simulink model "Power_Control"  (R2023b)
settings: Solver=FixedStepAuto  StartTime=0.0  StopTime=0.225  RelTol=1e-3
libraries: simulink x1
settings Model: Creator=no  LastModifiedBy=joser
settings OptimizationCC: DefaultParameterBehavior=Inlined
settings RTWCC: Description=INTECRIO Real-Time Target  SystemTargetFile=irt.tlc  TemplateMakefile=irt_default_tmf
settings STFCustomTargetCC: UtilityFuncGeneration=Shared location  MatFileLogging=on  GRTInterface=on  SystemTargetFile=irt.tlc
settings GRTTargetCC: UtilityFuncGeneration=Shared location  ParMdlRefBuildCompliant=off  CompOptLevelCompliant=off  ConcurrentExecutionCompliant=off  CombineOutputUpdateFcns=off  CPPClassGenCompliant=off  GRTInterface=on  UseToolchainInfoCompliant=off  GenerateASAP2=on

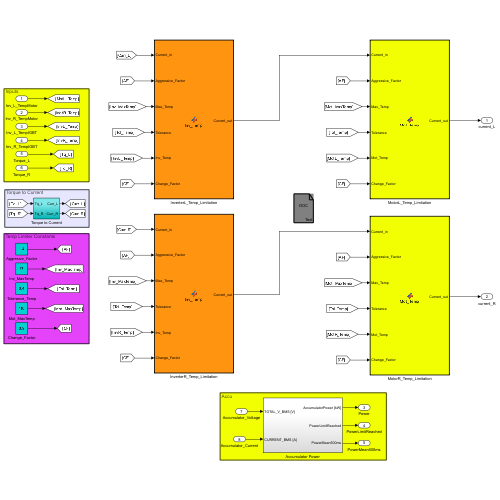
[thumbnail: Simulink's stored preview of the top-level diagram]
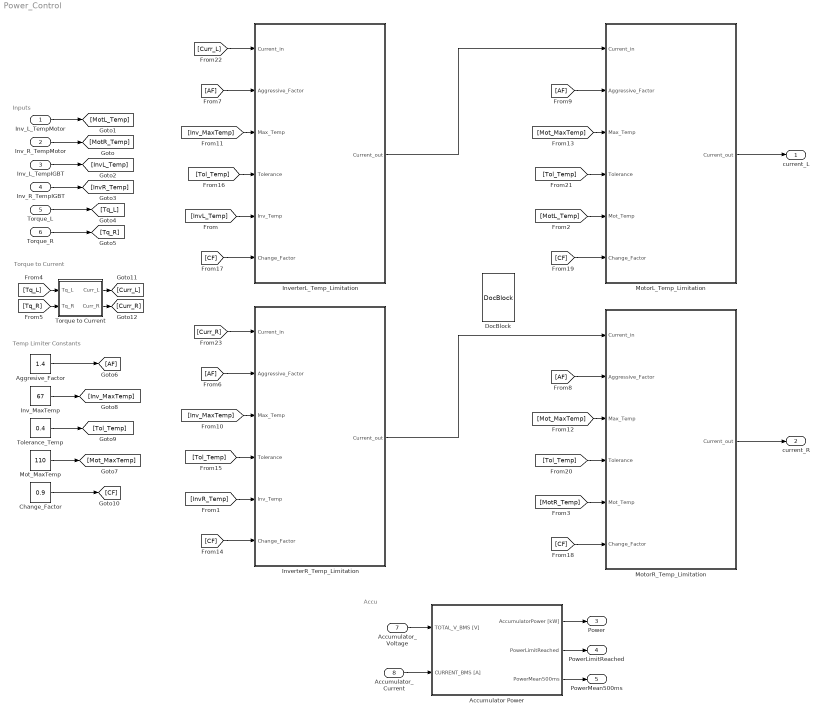
== system Power_Control ==
  note: Torque to Current
  note: Inputs
  note: Temp Limiter Constants
  note: Accu
  Inv_L_TempMotor : Inport
  Inv_R_TempMotor : Inport  Port=2
  Inv_L_TempIGBT : Inport  Port=3
  Inv_R_TempIGBT : Inport  Port=4
  Torque_L : Inport  Port=5
  Torque_R : Inport  Port=6
  Accumulator_Voltage : Inport  Port=7
  Accumulator_Current : Inport  Port=8
  Accumulator Power : Subsystem
  Aggresive_Factor : Constant  Value=1.4
  Change_Factor : Constant  Value=0.9
  DocBlock : simulink/Model-Wide Utilities/DocBlock  DocumentType=Text
      content=|
      | ------------------------ POWER CONTROL FUNCTIONS --------------------------
      |
      | Current_in -> Input current (A). The inverter has 0.001A of resolution.
      |
      | Current_out -> Output current (A)
      |
      | Aggressive_Factor -> Initial Aggressive Factor Value expressed as a percentage (%)
      | This value affects the aggressiveness of all temperature limitations, especially the
      | first one (when the algorithm starts to limit). This factor actuates on all limitations,
      | it is the most important one
      |
      | Max_Temp -> Maximum allowed temperature (ºC)
      |
      | Tolerance -> Tolerance for temperature range (ºC)
      |
      | Inv_Temp/Mot_Temp -> Actual Motors or Inverters temperature (ºC)
      |
      | Change_Factor -> Change Factor for adjusting aggressiveness, expressed as a percentage (%)
      | This value affects the aggressiveness starting from the second temperature limitation (when
      | already has started limiting, then actuates). It is more aggressive than the aggressive factor,
      | but does not affects
      |
      | ------------------------ TORQUE to CURRENT --------------------------------
      |
      | Conversion obtained empirically.
      |
      | Tq_em -> The ETAS' Torque output.
      |
      | Tq_em = (3/2) x pp x (i_q x lambda + (L_d-L_q) x i_d x i_q)
      |
      | i_d = 0, we only command i_q. Then:
      |
      | i_q = Tq_em x (2/3) / (pp x lambda). With our parameters (talk to powertrain):
      |
      | i_q = Tq_em * 3.29 (SEND RMS CURRENT TO THE BAMOCAR!!!!)
  Inv_MaxTemp : Constant  Value=67
  InverterL_Temp_Limitation : MATLAB Function  TreatAsAtomicUnit=on
  InverterR_Temp_Limitation : MATLAB Function  TreatAsAtomicUnit=on
  Mot_MaxTemp : Constant  Value=110
  MotorL_Temp_Limitation : MATLAB Function  TreatAsAtomicUnit=on
  MotorR_Temp_Limitation : MATLAB Function  TreatAsAtomicUnit=on
  Tolerance_Temp : Constant  Value=0.4
  Torque to Current : Subsystem
  current_L : Outport
  current_R : Outport  Port=2
  Power : Outport  Port=3  VectorParamsAs1DForOutWhenUnconnected=off
  PowerLimitReached : Outport  Port=4  VectorParamsAs1DForOutWhenUnconnected=off
  PowerMean500ms : Outport  Port=5  VectorParamsAs1DForOutWhenUnconnected=off
  wires:
  Inv_R_TempMotor/1 -> [MotR_Temp]
  Inv_L_TempMotor/1 -> [MotL_Temp]
  Inv_L_TempIGBT/1 -> [InvL_Temp]
  Inv_R_TempIGBT/1 -> [InvR_Temp]
  Torque_R/1 -> [Tq_R]
  Torque_L/1 -> [Tq_L]
  Change_Factor/1 -> [CF]
  Mot_MaxTemp/1 -> [Mot_MaxTemp]
  Tolerance_Temp/1 -> [Tol_Temp]
  Inv_MaxTemp/1 -> [Inv_MaxTemp]
  Aggresive_Factor/1 -> [AF]
  [MotL_Temp] -> MotorL_Temp_Limitation/5(Mot_Temp)
  [MotR_Temp] -> MotorR_Temp_Limitation/5(Mot_Temp)
  [InvL_Temp] -> InverterL_Temp_Limitation/5(Inv_Temp)
  [InvR_Temp] -> InverterR_Temp_Limitation/5(Inv_Temp)
  [Curr_L] -> InverterL_Temp_Limitation/1(Current_in)
  [Curr_R] -> InverterR_Temp_Limitation/1(Current_in)
  [AF] -> InverterR_Temp_Limitation/2(Aggressive_Factor)
  [AF] -> InverterL_Temp_Limitation/2(Aggressive_Factor)
  [AF] -> MotorL_Temp_Limitation/2(Aggressive_Factor)
  [AF] -> MotorR_Temp_Limitation/2(Aggressive_Factor)
  [Inv_MaxTemp] -> InverterL_Temp_Limitation/3(Max_Temp)
  [Inv_MaxTemp] -> InverterR_Temp_Limitation/3(Max_Temp)
  [Mot_MaxTemp] -> MotorR_Temp_Limitation/3(Max_Temp)
  [Mot_MaxTemp] -> MotorL_Temp_Limitation/3(Max_Temp)
  [Tol_Temp] -> InverterR_Temp_Limitation/4(Tolerance)
  [Tol_Temp] -> InverterL_Temp_Limitation/4(Tolerance)
  [CF] -> InverterL_Temp_Limitation/6(Change_Factor)
  [CF] -> InverterR_Temp_Limitation/6(Change_Factor)
  [CF] -> MotorL_Temp_Limitation/6(Change_Factor)
  [CF] -> MotorR_Temp_Limitation/6(Change_Factor)
  [Tol_Temp] -> MotorL_Temp_Limitation/4(Tolerance)
  [Tol_Temp] -> MotorR_Temp_Limitation/4(Tolerance)
  InverterR_Temp_Limitation/1(Current_out) -> MotorR_Temp_Limitation/1(Current_in)
  InverterL_Temp_Limitation/1(Current_out) -> MotorL_Temp_Limitation/1(Current_in)
  Accumulator_Voltage/1 -> Accumulator Power/1(TOTAL_V_BMS [V])
  Accumulator_Current/1 -> Accumulator Power/2(CURRENT_BMS [A])
  Accumulator Power/1(AccumulatorPower [kW]) -> Power/1
  Accumulator Power/3(PowerMean500ms) -> PowerMean500ms/1
  Accumulator Power/2(PowerLimitReached) -> PowerLimitReached/1
  [Tq_L] -> Torque to Current/1(Tq_L)
  [Tq_R] -> Torque to Current/2(Tq_R)
  Torque to Current/1(Curr_L) -> [Curr_L]
  Torque to Current/2(Curr_R) -> [Curr_R]
  MotorL_Temp_Limitation/1(Current_out) -> current_L/1
  MotorR_Temp_Limitation/1(Current_out) -> current_R/1

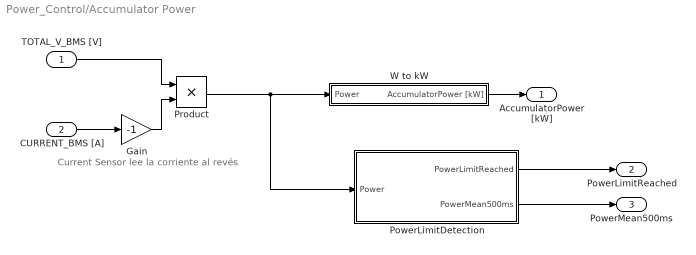
== system Power_Control/Accumulator Power ==
  note: Current Sensor lee la corriente al revés
  TOTAL_V_BMS [V] : Inport
  CURRENT_BMS [A] : Inport  Port=2
  Gain : Gain  Gain=-1
  PowerLimitDetection : Subsystem  TreatAsAtomicUnit=on
  Product : Product
  W to kW : Subsystem
  AccumulatorPower [kW] : Outport  VectorParamsAs1DForOutWhenUnconnected=off
  PowerLimitReached : Outport  Port=2  VectorParamsAs1DForOutWhenUnconnected=off
  PowerMean500ms : Outport  Port=3  VectorParamsAs1DForOutWhenUnconnected=off
  wires:
  Product/1 -> W to kW/1(Power), PowerLimitDetection/1(Power)
  PowerLimitDetection/1(PowerLimitReached) -> PowerLimitReached/1
  PowerLimitDetection/2(PowerMean500ms) -> PowerMean500ms/1
  TOTAL_V_BMS [V]/1 -> Product/1
  CURRENT_BMS [A]/1 -> Gain/1
  W to kW/1(AccumulatorPower [kW]) -> AccumulatorPower [kW]/1
  Gain/1 -> Product/2

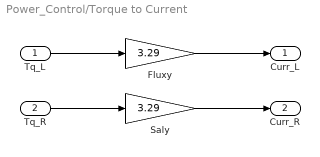
== system Power_Control/Torque to Current ==
  Tq_L : Inport
  Tq_R : Inport  Port=2
  Fluxy : Gain  Gain=3.29
  Saly : Gain  Gain=3.29
  Curr_L : Outport
  Curr_R : Outport  Port=2
  wires:
  Tq_L/1 -> Fluxy/1
  Tq_R/1 -> Saly/1
  Fluxy/1 -> Curr_L/1
  Saly/1 -> Curr_R/1

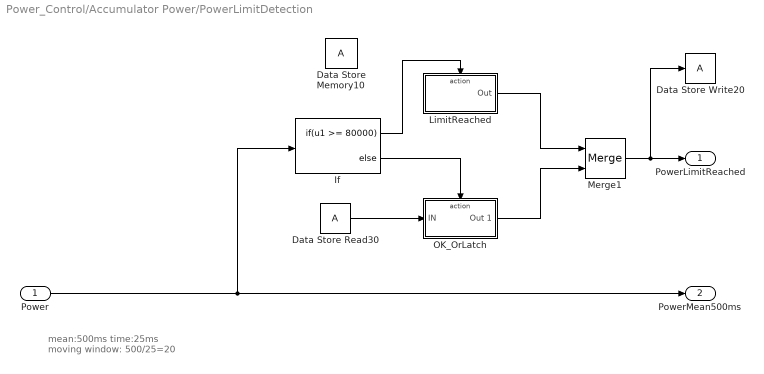
== system Power_Control/Accumulator Power/PowerLimitDetection ==
  note: mean:500ms
      | time:25ms
      | moving window: 500/25=20
  Power : Inport
  Data Store Memory10 : DataStoreMemory  ReadBeforeWriteMsg=warning  WriteAfterWriteMsg=warning  WriteAfterReadMsg=warning  ShowAdditionalParam=off
  Data Store Read30 : DataStoreRead  IndexOptions=Index vector (dialog)  Indices=1  OutputSizes=1
  Data Store Write20 : DataStoreWrite  IndexOptions=Index vector (dialog)  Indices=1  OutputSizes=1
  If : If  IfExpression=u1 >= 80000
  LimitReached : Subsystem  TreatAsAtomicUnit=on
  Merge1 : Merge
  OK_OrLatch : Subsystem  TreatAsAtomicUnit=on
  PowerLimitReached : Outport  VectorParamsAs1DForOutWhenUnconnected=off
  PowerMean500ms : Outport  Port=2  VectorParamsAs1DForOutWhenUnconnected=off
  wires:
  Power/1 -> If/1, PowerMean500ms/1
  If/1 -> LimitReached/Action
  If/2 -> OK_OrLatch/Action
  LimitReached/1("Out ") -> Merge1/1
  OK_OrLatch/1(Out 1) -> Merge1/2
  Merge1/1 -> Data Store Write20/1, PowerLimitReached/1
  Data Store Read30/1 -> OK_OrLatch/1(IN)

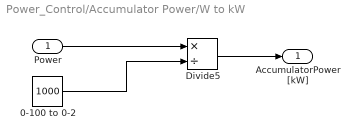
== system Power_Control/Accumulator Power/W to kW ==
  Power : Inport
  0-100 to 0-2 : Constant  Value=1000
  Divide5 : Product  Inputs=*/
  AccumulatorPower [kW] : Outport  VectorParamsAs1DForOutWhenUnconnected=off
  wires:
  Power/1 -> Divide5/1
  0-100 to 0-2/1 -> Divide5/2
  Divide5/1 -> AccumulatorPower [kW]/1

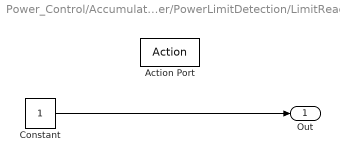
== system Power_Control/Accumulator Power/PowerLimitDetection/LimitReached ==
  Action Port : ActionPort  ActionPortLabel=if(u1 >= 80000)
  Constant : Constant
  "Out " : Outport  VectorParamsAs1DForOutWhenUnconnected=off
  wires:
  Constant/1 -> "Out "/1

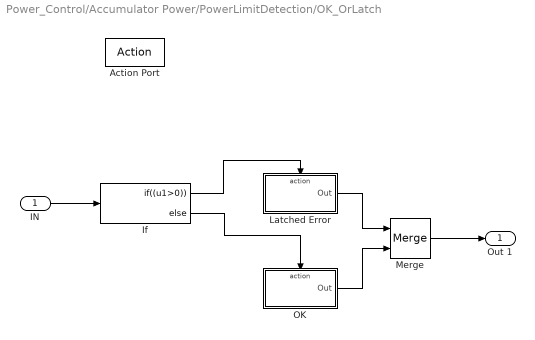
== system Power_Control/Accumulator Power/PowerLimitDetection/OK_OrLatch ==
  IN : Inport
  Action Port : ActionPort  ActionPortLabel=else
  If : If  IfExpression=(u1>0)
  Latched Error : Subsystem  TreatAsAtomicUnit=on
  Merge : Merge
  OK : Subsystem  TreatAsAtomicUnit=on
  Out 1 : Outport  VectorParamsAs1DForOutWhenUnconnected=off
  wires:
  IN/1 -> If/1
  If/1 -> Latched Error/Action
  If/2 -> OK/Action
  Latched Error/1("Out ") -> Merge/1
  OK/1("Out ") -> Merge/2
  Merge/1 -> Out 1/1

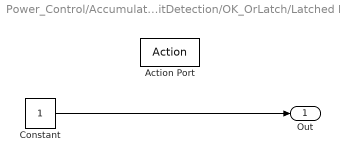
== system Power_Control/Accumulator Power/PowerLimitDetection/OK_OrLatch/Latched Error ==
  Action Port : ActionPort  ActionPortLabel=if((u1>0))
  Constant : Constant
  "Out " : Outport  VectorParamsAs1DForOutWhenUnconnected=off
  wires:
  Constant/1 -> "Out "/1

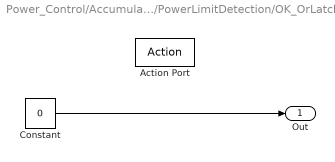
== system Power_Control/Accumulator Power/PowerLimitDetection/OK_OrLatch/OK ==
  Action Port : ActionPort  ActionPortLabel=else
  Constant : Constant  Value=0
  "Out " : Outport  VectorParamsAs1DForOutWhenUnconnected=off
  wires:
  Constant/1 -> "Out "/1

== matlab function Power_Control/MotorR_Temp_Limitation ==
  data: Current_in input; Aggressive_Factor input; Max_Temp input; Current_out output; Tolerance input; Mot_Temp input; Change_Factor input
function Current_out = Mot_Temp(Current_in, Aggressive_Factor, Max_Temp, Tolerance, Mot_Temp, Change_Factor)
%% Initializing internal variables
% If they have not been defined yet, initiate them

    % Last_Temp (ºC) -> Mot_Temp of the last iteration
    persistent Last_Temp
    if isempty(Last_Temp)
        Last_Temp = 0;
    end

    % Aggressive Factor Value (%) -> Factor of Current reduction. Changes
    % every iteration due to counters, but can be reset if the Mot_Temp is
    % acceptable
    persistent AF_Value
    if isempty(AF_Value)
        AF_Value = Aggressive_Factor;
    end

    % Times_Incremented -> Counter of the Temp_Change higher than Tolerance
    persistent Times_Incremented
    if isempty(Times_Incremented)
        Times_Incremented = 1;
    end

    % Times_Decremented -> Counter of the Temp_Change lower than -Tolerance
    persistent Times_Decremented
    if isempty(Times_Decremented)
        Times_Decremented = 1;
    end

%% Derivative
    % Compute the Temperature difference between the last temp and the
    % actual one
Temp_Change = Mot_Temp - Last_Temp;

%% Temperature Control Logic
    
    if (Temp_Change > Tolerance)
        % Temperature is increasing beyond Tolerance, limit the Current
        % more aggressively to reduce the Mot_Temp
        New_Current = Current_in * (1 - (AF_Value * Temp_Change / 100));
        % Increase the Aggresive Factor for the next iteration and sum 1 to
        % the Increment counter
        AF_Value = AF_Value + (Change_Factor * Times_Incremented);
        Times_Incremented = Times_Incremented + 1;
        Times_Decremented = 1;

    elseif (Temp_Change < -Tolerance)
        % Temperature is cooling down beyond Tolerance, allow to normalize
        % the Current (then the temperature rises)
        New_Current = Current_in * (1 - (AF_Value * Temp_Change / 100));
        % Decrease the Aggressive Factor for the next iteration and sum 1
        % to the Decrement counter
        AF_Value = AF_Value - (Change_Factor * Times_Decremented);
        Times_Incremented = 1;
        Times_Decremented = Times_Decremented + 1;

    else
        % Temperature is stable (within Tolerance), gradually reduce Current
        New_Current = Current_in * (1 - AF_Value / 10);
        % Reset both counters
        Times_Incremented = 1;
        Times_Decremented = 1;

    end
%% Compare the Actual Current with the New Current

    if (((New_Current > Current_in) && (Current_in >= 0)) || ((New_Current < Current_in) && (Current_in < 0)))
        % Ensure the New_Current does not exceed the input current when accelerating
        % If regen, then the New_Current cannot be lower than the Current_in, it
        % has to be higher (they are both negative)
        New_Current = Current_in;

    elseif (sign(New_Current) ~= sign(Current_in))
        % If it was demanding a positive current, but New_Current is
        % negative, just output 0 (so we do not regenerate when we don't
        % want). Same for the inverse case
        New_Current = 0;
        
    end

%% Output values

    if (Mot_Temp > Max_Temp)
        % If the Mot_Temp is higher than the Maximum_Temp selected, limit
        % the Current with the calculated one
        Current_out = New_Current;

    else
        % If the Mot_Temp is acceptable, maintain the current demanded and
        % do not apply the calculated Aggresive Factor Value
        Current_out = Current_in;
        AF_Value = Aggressive_Factor;

    end
% Update the last known Temperature
Last_Temp = Mot_Temp;
end

== matlab function Power_Control/InverterL_Temp_Limitation ==
  data: Current_in input; Aggressive_Factor input; Max_Temp input; Current_out output; Tolerance input; Inv_Temp input; Change_Factor input
function Current_out = Inv_Temp(Current_in, Aggressive_Factor, Max_Temp, Tolerance, Inv_Temp, Change_Factor)
%% Initializing internal variables
% If they have not been defined yet, initiate them

    % Last_Temp (ºC) -> Inv_Temp of the last iteration
    persistent Last_Temp
    if isempty(Last_Temp)
        Last_Temp = 0;
    end

    % Aggressive Factor Value (%) -> Factor of Current reduction. Changes
    % every iteration due to counters, but can be reset if the Inv_Temp is
    % acceptable
    persistent AF_Value
    if isempty(AF_Value)
        AF_Value = Aggressive_Factor;
    end

    % Times_Incremented -> Counter of the Temp_Change higher than Tolerance
    persistent Times_Incremented
    if isempty(Times_Incremented)
        Times_Incremented = 1;
    end

    % Times_Decremented -> Counter of the Temp_Change lower than -Tolerance
    persistent Times_Decremented
    if isempty(Times_Decremented)
        Times_Decremented = 1;
    end

%% Derivative
    % Compute the Temperature difference between the last temp and the
    % actual one
Temp_Change = Inv_Temp - Last_Temp;

%% Temperature Control Logic
    
    if (Temp_Change > Tolerance)
        % Temperature is increasing beyond Tolerance, limit the Current
        % more aggressively to reduce the Inv_Temp
        New_Current = Current_in * (1 - (AF_Value * Temp_Change / 100));
        % Increase the Aggresive Factor for the next iteration and sum 1 to
        % the Increment counter
        AF_Value = AF_Value + (Change_Factor * Times_Incremented);
        Times_Incremented = Times_Incremented + 1;
        Times_Decremented = 1;

    elseif (Temp_Change < -Tolerance)
        % Temperature is cooling down beyond Tolerance, allow to normalize
        % the Current (then the temperature rises)
        New_Current = Current_in * (1 - (AF_Value * Temp_Change / 100));
        % Decrease the Aggressive Factor for the next iteration and sum 1
        % to the Decrement counter
        AF_Value = AF_Value - (Change_Factor * Times_Decremented);
        Times_Incremented = 1;
        Times_Decremented = Times_Decremented + 1;

    else
        % Temperature is stable (within Tolerance), gradually reduce Current
        New_Current = Current_in * (1 - AF_Value / 10);
        % Reset both counters
        Times_Incremented = 1;
        Times_Decremented = 1;

    end
%% Compare the Actual Current with the New Current

    if (((New_Current > Current_in) && (Current_in >= 0)) || ((New_Current < Current_in) && (Current_in < 0)))
        % Ensure the New_Current does not exceed the input current when accelerating
        % If regen, then the New_Current cannot be lower than the Current_in, it
        % has to be higher (they are both negative)
        New_Current = Current_in;

    elseif (sign(New_Current) ~= sign(Current_in))
        % If it was demanding a positive current, but New_Current is
        % negative, just output 0 (so we do not regenerate when we don't
        % want). Same for the inverse case
        New_Current = 0;
        
    end

%% Output values

    if (Inv_Temp > Max_Temp)
        % If the Inv_Temp is higher than the Maximum_Temp selected, limit
        % the Current with the calculated one
        Current_out = New_Current;

    else
        % If the Inv_Temp is acceptable, maintain the current demanded and
        % do not apply the calculated Aggresive Factor Value
        Current_out = Current_in;
        AF_Value = Aggressive_Factor;

    end
% Update the last known Temperature
Last_Temp = Inv_Temp;
end

== matlab function Power_Control/MotorL_Temp_Limitation ==
  data: Current_in input; Aggressive_Factor input; Max_Temp input; Current_out output; Tolerance input; Mot_Temp input; Change_Factor input
function Current_out = Mot_Temp(Current_in, Aggressive_Factor, Max_Temp, Tolerance, Mot_Temp, Change_Factor)
%% Initializing internal variables
% If they have not been defined yet, initiate them

    % Last_Temp (ºC) -> Mot_Temp of the last iteration
    persistent Last_Temp
    if isempty(Last_Temp)
        Last_Temp = 0;
    end

    % Aggressive Factor Value (%) -> Factor of Current reduction. Changes
    % every iteration due to counters, but can be reset if the Mot_Temp is
    % acceptable
    persistent AF_Value
    if isempty(AF_Value)
        AF_Value = Aggressive_Factor;
    end

    % Times_Incremented -> Counter of the Temp_Change higher than Tolerance
    persistent Times_Incremented
    if isempty(Times_Incremented)
        Times_Incremented = 1;
    end

    % Times_Decremented -> Counter of the Temp_Change lower than -Tolerance
    persistent Times_Decremented
    if isempty(Times_Decremented)
        Times_Decremented = 1;
    end

%% Derivative
    % Compute the Temperature difference between the last temp and the
    % actual one
Temp_Change = Mot_Temp - Last_Temp;

%% Temperature Control Logic
    
    if (Temp_Change > Tolerance)
        % Temperature is increasing beyond Tolerance, limit the Current
        % more aggressively to reduce the Mot_Temp
        New_Current = Current_in * (1 - (AF_Value * Temp_Change / 100));
        % Increase the Aggresive Factor for the next iteration and sum 1 to
        % the Increment counter
        AF_Value = AF_Value + (Change_Factor * Times_Incremented);
        Times_Incremented = Times_Incremented + 1;
        Times_Decremented = 1;

    elseif (Temp_Change < -Tolerance)
        % Temperature is cooling down beyond Tolerance, allow to normalize
        % the Current (then the temperature rises)
        New_Current = Current_in * (1 - (AF_Value * Temp_Change / 100));
        % Decrease the Aggressive Factor for the next iteration and sum 1
        % to the Decrement counter
        AF_Value = AF_Value - (Change_Factor * Times_Decremented);
        Times_Incremented = 1;
        Times_Decremented = Times_Decremented + 1;

    else
        % Temperature is stable (within Tolerance), gradually reduce Current
        New_Current = Current_in * (1 - AF_Value / 10);
        % Reset both counters
        Times_Incremented = 1;
        Times_Decremented = 1;

    end
%% Compare the Actual Current with the New Current

    if (((New_Current > Current_in) && (Current_in >= 0)) || ((New_Current < Current_in) && (Current_in < 0)))
        % Ensure the New_Current does not exceed the input current when accelerating
        % If regen, then the New_Current cannot be lower than the Current_in, it
        % has to be higher (they are both negative)
        New_Current = Current_in;

    elseif (sign(New_Current) ~= sign(Current_in))
        % If it was demanding a positive current, but New_Current is
        % negative, just output 0 (so we do not regenerate when we don't
        % want). Same for the inverse case
        New_Current = 0;
        
    end

%% Output values

    if (Mot_Temp > Max_Temp)
        % If the Mot_Temp is higher than the Maximum_Temp selected, limit
        % the Current with the calculated one
        Current_out = New_Current;

    else
        % If the Mot_Temp is acceptable, maintain the current demanded and
        % do not apply the calculated Aggresive Factor Value
        Current_out = Current_in;
        AF_Value = Aggressive_Factor;

    end
% Update the last known Temperature
Last_Temp = Mot_Temp;
end

== matlab function Power_Control/InverterR_Temp_Limitation ==
  data: Current_in input; Aggressive_Factor input; Max_Temp input; Current_out output; Tolerance input; Inv_Temp input; Change_Factor input
function Current_out = Inv_Temp(Current_in, Aggressive_Factor, Max_Temp, Tolerance, Inv_Temp, Change_Factor)
%% Initializing internal variables
% If they have not been defined yet, initiate them

    % Last_Temp (ºC) -> Inv_Temp of the last iteration
    persistent Last_Temp
    if isempty(Last_Temp)
        Last_Temp = 0;
    end

    % Aggressive Factor Value (%) -> Factor of Current reduction. Changes
    % every iteration due to counters, but can be reset if the Inv_Temp is
    % acceptable
    persistent AF_Value
    if isempty(AF_Value)
        AF_Value = Aggressive_Factor;
    end

    % Times_Incremented -> Counter of the Temp_Change higher than Tolerance
    persistent Times_Incremented
    if isempty(Times_Incremented)
        Times_Incremented = 1;
    end

    % Times_Decremented -> Counter of the Temp_Change lower than -Tolerance
    persistent Times_Decremented
    if isempty(Times_Decremented)
        Times_Decremented = 1;
    end

%% Derivative
    % Compute the Temperature difference between the last temp and the
    % actual one
Temp_Change = Inv_Temp - Last_Temp;

%% Temperature Control Logic
    
    if (Temp_Change > Tolerance)
        % Temperature is increasing beyond Tolerance, limit the Current
        % more aggressively to reduce the Inv_Temp
        New_Current = Current_in * (1 - (AF_Value * Temp_Change / 100));
        % Increase the Aggresive Factor for the next iteration and sum 1 to
        % the Increment counter
        AF_Value = AF_Value + (Change_Factor * Times_Incremented);
        Times_Incremented = Times_Incremented + 1;
        Times_Decremented = 1;

    elseif (Temp_Change < -Tolerance)
        % Temperature is cooling down beyond Tolerance, allow to normalize
        % the Current (then the temperature rises)
        New_Current = Current_in * (1 - (AF_Value * Temp_Change / 100));
        % Decrease the Aggressive Factor for the next iteration and sum 1
        % to the Decrement counter
        AF_Value = AF_Value - (Change_Factor * Times_Decremented);
        Times_Incremented = 1;
        Times_Decremented = Times_Decremented + 1;

    else
        % Temperature is stable (within Tolerance), gradually reduce Current
        New_Current = Current_in * (1 - AF_Value / 10);
        % Reset both counters
        Times_Incremented = 1;
        Times_Decremented = 1;

    end
%% Compare the Actual Current with the New Current

    if (((New_Current > Current_in) && (Current_in >= 0)) || ((New_Current < Current_in) && (Current_in < 0)))
        % Ensure the New_Current does not exceed the input current when accelerating
        % If regen, then the New_Current cannot be lower than the Current_in, it
        % has to be higher (they are both negative)
        New_Current = Current_in;

    elseif (sign(New_Current) ~= sign(Current_in))
        % If it was demanding a positive current, but New_Current is
        % negative, just output 0 (so we do not regenerate when we don't
        % want). Same for the inverse case
        New_Current = 0;
        
    end

%% Output values

    if (Inv_Temp > Max_Temp)
        % If the Inv_Temp is higher than the Maximum_Temp selected, limit
        % the Current with the calculated one
        Current_out = New_Current;

    else
        % If the Inv_Temp is acceptable, maintain the current demanded and
        % do not apply the calculated Aggresive Factor Value
        Current_out = Current_in;
        AF_Value = Aggressive_Factor;

    end
% Update the last known Temperature
Last_Temp = Inv_Temp;
end
